simulink model "controller_3dof"  (R2023a)
settings: Solver=FixedStepAuto  StartTime=0.0  StopTime=inf  FixedStep=0.01  RelTol=1e-3  EnableMultiTasking=on
values from neighbouring files (symbols this model uses):
  mf = [22602; 0; -42062;]    [main_3dof.m]
  P0 = diag([P0_ph_meas,P0_th_meas,P0_ps_meas,P0_bias_wp,P0_bias_wq,P0_bias_wr])    [main_3dof.m]
  param = [Ixx;Iyy;Izz;l;k;b;m]    [main_3dof.m]
  Q = diag([q_angle,q_angle,q_angle, q_bias_w_b,q_bias_w_b,q_bias_w_b])    [main_3dof.m]
  R = diag([r_th_meas,r_th_meas,r_ps_meas])    [main_3dof.m]
  Rbody_frd = [cos(angleZ) -sin(angleZ)   0 ... (first row only)    [main_3dof.m]
  Rbody_ned = Rbody_frd*Rfrd_ned    [main_3dof.m]
  Ts_EKF_integr = 0.01    [main_3dof.m]
  Ts_EKF_meas = 0.05    [main_3dof.m]
  Ts_slk = 0.01    [main.m]    (also in main_3dof.m)
  x0EKF = [ph0;th0;ps0;bias_wp0;bias_wq0;bias_wr0]    [main_3dof.m]
undefined symbols (not defined in the file or in its folder): dev, DiscIntNeverNeededParam, Kv, Kx, Main, pwm_output0
libraries: px4Sensorslib x4, px4lib x1, px4uORBlib x1
settings Model: SimulationMode=external  ExtModeTrigDuration=10  Creator=ArriGE66  LastModifiedBy=User
settings SolverCC: PositivePriorityOrder=on
settings OptimizationCC: EnhancedBackFolding=on  PassReuseOutputArgsAs=Individual arguments  ZeroExternalMemoryAtStartup=off  ZeroInternalMemoryAtStartup=off  MaxStackSize=64  OptimizeBlockOrder=speed  DifferentSizesBufferReuse=on  OptimizationCustomize=off  EfficientTunableParamExpr=on
settings DebuggingCC: ParameterTunabilityLossMsg=error
settings HardwareCC: ProdBitPerPointer=32  ProdBitPerSizeT=32  ProdBitPerPtrDiffT=32  ProdLargestAtomicInteger=Long  ProdLargestAtomicFloat=Double  ProdWordSize=32  ProdLongLongMode=on  ProdHWDeviceType=ARM Compatible->ARM Cortex
settings SFSimCC: MATLABDynamicMemAlloc=off  SimTargetLang=C++
settings RTWCC: Description=Embedded Coder  SystemTargetFile=ert.tlc  HardwareBoard=PX4 Cube Orange  TemplateMakefile=ert_default_tmf  Toolchain=GNU Tools for PX4 Autopilots  TargetLang=C++
settings CodeAppCC: ForceParamTrailComments=on  IgnoreCustomStorageClasses=off  OperatorAnnotations=on  SimulinkDataObjDesc=on  SFDataObjDesc=on  InsertBlockDesc=on
settings ERTTargetCC: ExtMode=on  ExtModeTransport=3  ExtModeStaticAlloc=on  ExtModeStaticAllocSize=1024  ExtModeMexFile=ext_xcp  ExtModeMexArgs=1 COM10 3000000  ExtModeIntrfLevel=Level2 - Open

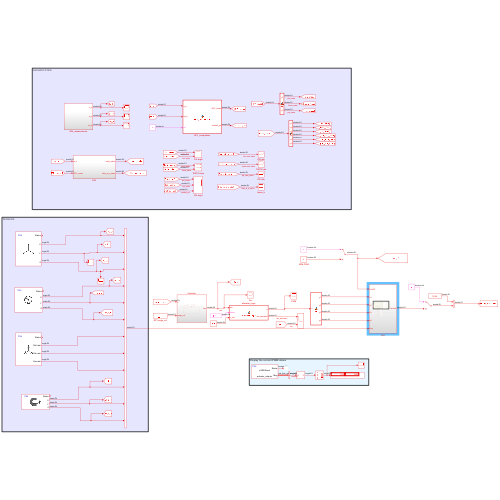
[thumbnail: Simulink's stored preview of the top-level diagram]
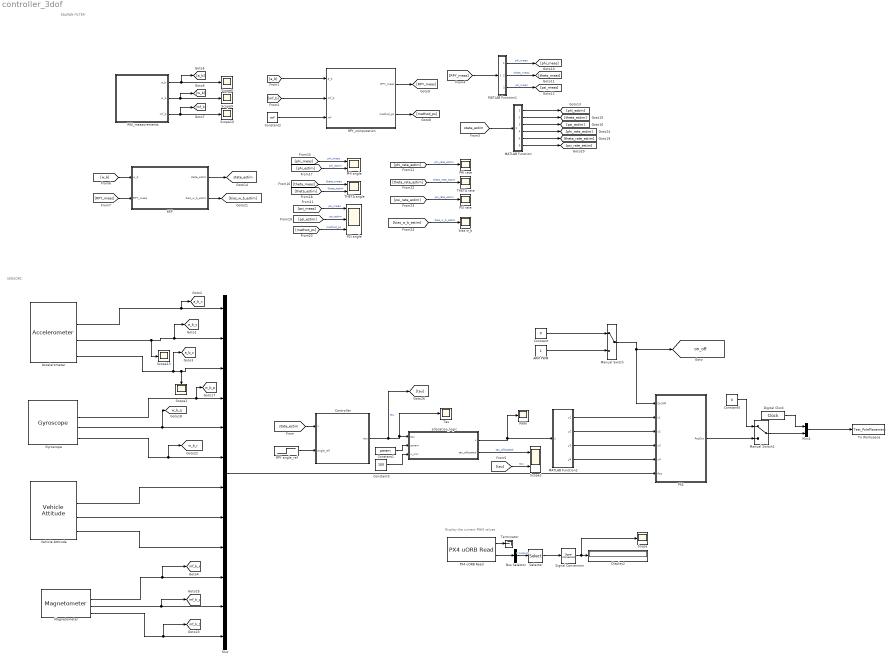
== system controller_3dof ==
  note: KALMAN FILTER
  note: SENSORS
  note: Display the current PWM values
  ARM PWM : Constant  OutDataTypeStr=boolean  SampleTime=0.01
  Accelerometer : px4Sensorslib/Accelerometer  uorbTimeStamp=off  BlockingMode=off  BlockTimeout=1e-3  sampleTime=1/100
  Bus Selector : BusSelector  OutputSignals=output
  Constant : Constant  Value=0  OutDataTypeStr=boolean
  Constant1 : Constant  Value=param
  Constant2 : Constant  Value=mf
  Constant3 : Constant  Value=100  SampleTime=0.01
  Constant5 : Constant  Value=0  OutDataTypeStr=boolean
  Controller : Subsystem
  Digital Clock : DigitalClock  SampleTime=0.01
  Display2 : Display
  EKF : Subsystem
  Gyroscope : px4Sensorslib/Gyroscope  uorbTimeStamp=off  BlockingMode=off  BlockTimeout=1e-3  sampleTime=1/100
  IMU_measurements : Subsystem
  MATLAB Function : MATLAB Function  TreatAsAtomicUnit=on
  MATLAB Function1 : MATLAB Function  TreatAsAtomicUnit=on
  MATLAB Function2 : MATLAB Function  TreatAsAtomicUnit=on
  Magnetometer : px4Sensorslib/Magnetometer  uorbTimeStamp=off  BlockingMode=off  BlockTimeout=1e-3  sampleTime=0.01
  Manual Switch : ManualSwitch
  Manual Switch1 : ManualSwitch
  Mux : Mux  Inputs=12
  Mux1 : Mux  Inputs=2
  PHI angle : Scope  NumInputPorts=2
  PHI rate : Scope
  PSI angle : Scope  NumInputPorts=3
  PSI rate : Scope
  PWM : Scope
  PX4 : Subsystem
  PX4 uORB Read : px4uORBlib/PX4 uORB Read  uORBTopic=actuator_outputs  selectInstance=actuator_outputs  SampleTime=0.01  BlockingMode=off  BlockTimeout=1e-3
  RPY angle_ref : Step  Time=0  After=zeros(3,1)  SampleTime=0.01
  RPY_computation : MATLAB Function  TreatAsAtomicUnit=on
  Scope{,1,8..10,13} (6 alike) : Scope
  Scope2 : Scope  NumInputPorts=2
  Selector : Selector  InputPortWidth=16  IndexOptions=Index vector (dialog)  Indices=[1 2]  OutputSizes=1
  Signal Conversion : SignalConversion  OverrideOpt=off
  THETA angle : Scope  NumInputPorts=2
  THETA rate : Scope
  Tau : Scope
  Terminator : Terminator
  To Workspace : ToWorkspace  VariableName=Test_PolePlacement  SampleTime=-1
      settings: Save2DSignal=2-D array (concatenate along first dimension)
  Vehicle Attitude : px4Sensorslib/Vehicle Attitude  rollRate=on  pitchRate=on  yawRate=on  quaternion=off  uorbTimeStamp=off  BlockingMode=off  BlockTimeout=0.001  sampleTime=1/100
  allocation_logic : MATLAB Function  TreatAsAtomicUnit=on
  bias w_b : Scope
  tag scope: a_b_x=global, a_b_y=global, a_b_z=global, mf_b_x=global, mf_b_y=global, mf_b_z=global, on_off=global, state_estim=global, w_b_p=global, w_b_q=global, w_b_r=global
  wires:
  Bus Selector/1 -> Selector/1  "<output>"
  PX4 uORB Read/1 -> Terminator/1
  Selector/1 -> Signal Conversion/1
  PX4 uORB Read/2 -> Bus Selector/1
  Signal Conversion/1 -> Scope/1, Display2/1
  Vehicle Attitude/3 -> Mux/8
  Vehicle Attitude/2 -> Mux/7
  ARM PWM/1 -> Manual Switch/2
  Constant/1 -> Manual Switch/1
  Gyroscope/4 -> [w_b_r], Mux/6
  Gyroscope/3 -> [w_b_q], Mux/5
  Gyroscope/2 -> [w_b_p], Mux/4
  Accelerometer/2 -> [a_b_x], Mux/1
  Accelerometer/3 -> Scope13/1, [a_b_y], Mux/2
  Accelerometer/4 -> [a_b_z], Mux/3, Scope1/1
  Constant5/1 -> Manual Switch1/1
  Mux1/1 -> To Workspace/1
  Digital Clock/1 -> Mux1/1
  Manual Switch1/1 -> Mux1/2
  Vehicle Attitude/4 -> Mux/9
  Magnetometer/2 -> [mf_b_x], Mux/10
  Magnetometer/3 -> [mf_b_y], Mux/11
  Magnetometer/4 -> [mf_b_z], Mux/12
  MATLAB Function1/2(y2) -> [theta_meas]  "theta_meas"
  [bias_w_b_estim] -> bias w_b/1  "bias_w_b_estim"
  [mf_b] -> RPY_computation/2(mf_b)
  [theta_estim] -> THETA angle/2  "theta_estim"
  MATLAB Function1/1(y1) -> [phi_meas]  "phi_meas"
  [RPY_meas] -> EKF/2(RPY_meas)
  [psi_meas] -> PSI angle/1  "psi_meas"
  [method_ps] -> PSI angle/3  "method_ps"
  IMU_measurements/2(w_b) -> Scope9/1, [w_b]
  [psi_estim] -> PSI angle/2  "psi_estim"
  MATLAB Function1/3(y3) -> [psi_meas]  "psi_meas"
  [RPY_meas] -> MATLAB Function1/1(u)
  [theta_meas] -> THETA angle/1  "theta_meas"
  [phi_rate_estim] -> PHI rate/1  "phi_rate_estim"
  [psi_rate_estim] -> PSI rate/1  "psi_rate_estim"
  [theta_rate_estim] -> THETA rate/1  "theta_rate_estim"
  EKF/1(state_estim) -> [state_estim]
  [phi_estim] -> PHI angle/2  "phi_estim"
  [w_b] -> EKF/1(w_b)
  IMU_measurements/3(mf_b) -> [mf_b], Scope10/1
  Constant2/1 -> RPY_computation/3(mf)
  IMU_measurements/1(a_b) -> [a_b], Scope8/1
  RPY_computation/2(method_ps) -> [method_ps]
  [a_b] -> RPY_computation/1(a_b)
  EKF/2(bias_w_b_estim) -> [bias_w_b_estim]
  [phi_meas] -> PHI angle/1  "phi_meas"
  RPY_computation/1(RPY_meas) -> [RPY_meas]
  Manual Switch/1 -> [on_off], PX4/1(On/Off)
  Mux/1 -> PX4/6(Acq)
  PX4/1(AcqOut) -> Manual Switch1/2
  [state_estim] -> MATLAB Function/1(u)
  MATLAB Function/1(y1) -> [phi_estim]
  MATLAB Function/2(y2) -> [theta_estim]
  MATLAB Function/3(y3) -> [psi_estim]
  MATLAB Function/4(y4) -> [phi_rate_estim]
  MATLAB Function/5(y5) -> [theta_rate_estim]
  MATLAB Function/6(y6) -> [psi_rate_estim]
  MATLAB Function2/4(y4) -> PX4/5(u4)
  MATLAB Function2/3(y3) -> PX4/4(u3)
  MATLAB Function2/2(y2) -> PX4/3(u2)
  MATLAB Function2/1(y1) -> PX4/2(u1)
  allocation_logic/2(tau_allocated) -> Scope2/1  "tau_allocated"
  allocation_logic/1(u) -> PWM/1, MATLAB Function2/1(u)
  Controller/1(tau) -> Tau/1, allocation_logic/1(tau), [tau]  "tau"
  RPY angle_ref/1 -> Controller/2(angle_ref)
  [tau] -> Scope2/2  "tau"
  Constant1/1 -> allocation_logic/2(param)
  [state_estim] -> Controller/1(x)
  Constant3/1 -> allocation_logic/3(u_min)

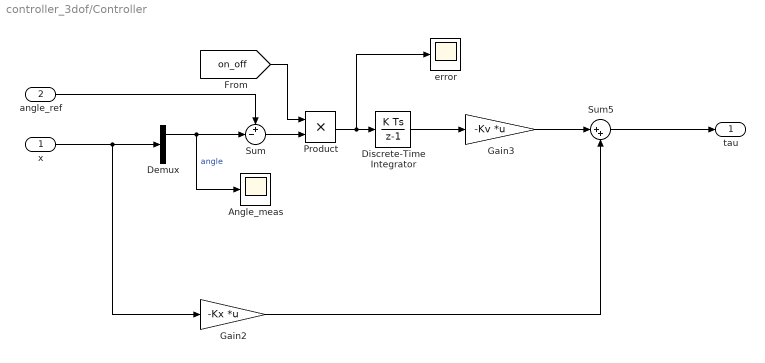
== system controller_3dof/Controller ==
  x : Inport
  angle_ref : Inport  Port=2
  Angle_meas : Scope
  Demux : Demux  Outputs=2
  Discrete-Time Integrator : DiscreteIntegrator  SampleTime=Ts_slk  ICPrevOutput=DiscIntNeverNeededParam  ICPrevScaledInput=DiscIntNeverNeededParam
  Gain2 : Gain  Gain=-Kx  Multiplication=Matrix(K*u)
  Gain3 : Gain  Gain=-Kv  Multiplication=Matrix(K*u)
  Product : Product
  Sum : Sum  Inputs=+-|
  Sum5 : Sum  Inputs=|++
  error : Scope
  tau : Outport
  wires:
  x/1 -> Gain2/1, Demux/1
  Sum5/1 -> tau/1
  angle_ref/1 -> Sum/1
  Discrete-Time Integrator/1 -> Gain3/1
  Gain3/1 -> Sum5/1
  Demux/1 -> Angle_meas/1, Sum/2  "angle"
  Gain2/1 -> Sum5/2
  Sum/1 -> Product/2
  [on_off] -> Product/1
  Product/1 -> error/1, Discrete-Time Integrator/1

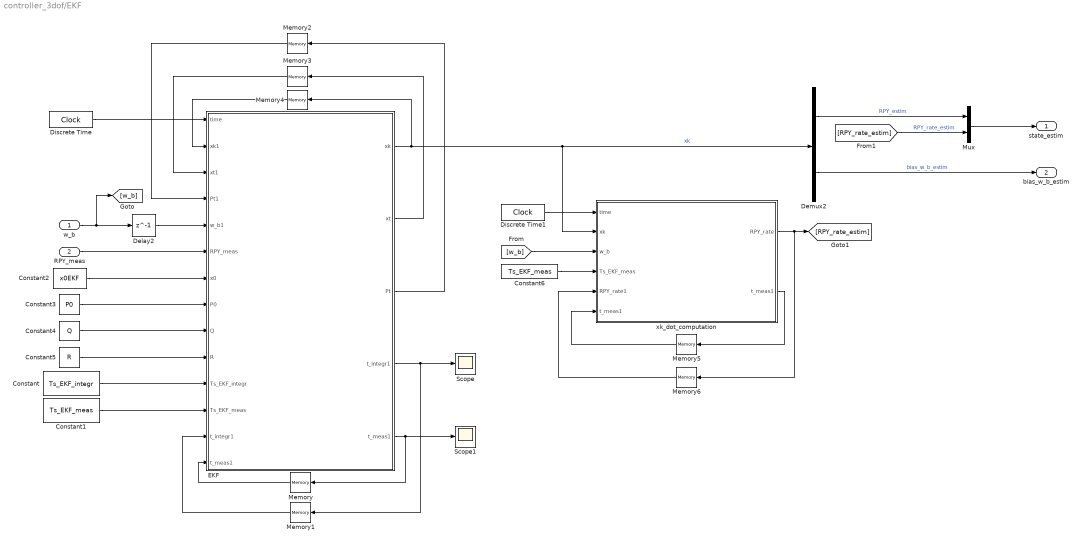
== system controller_3dof/EKF ==
  w_b : Inport
  RPY_meas : Inport  Port=2
  Constant : Constant  Value=Ts_EKF_integr
  Constant1 : Constant  Value=Ts_EKF_meas
  Constant2 : Constant  Value=x0EKF
  Constant3 : Constant  Value=P0
  Constant4 : Constant  Value=Q
  Constant5 : Constant  Value=R
  Constant6 : Constant  Value=Ts_EKF_meas
  Delay2 : Delay  DelayLength=1  SampleTime=Ts_EKF_integr
  Demux2 : Demux  Outputs=2
  Discrete Time : DigitalClock  SampleTime=Ts_slk
  Discrete Time1 : DigitalClock  SampleTime=Ts_slk
  EKF : MATLAB Function  TreatAsAtomicUnit=on
  Memory{,1..6} (7 alike) : Memory
  Mux : Mux  Inputs=2
  Scope : Scope
  Scope1 : Scope
  xk_dot_computation : MATLAB Function  TreatAsAtomicUnit=on
  state_estim : Outport
  bias_w_b_estim : Outport  Port=2
  wires:
  w_b/1 -> Delay2/1, [w_b]
  Constant4/1 -> EKF/9(Q)
  Constant2/1 -> EKF/7(x0)
  Constant5/1 -> EKF/10(R)
  Memory/1 -> EKF/14("t_meas1 ")
  EKF/2(xt) -> Memory3/1
  Memory2/1 -> EKF/4(Pt1)
  EKF/3(Pt) -> Memory2/1
  RPY_meas/1 -> EKF/6(RPY_meas)
  Discrete Time/1 -> EKF/1(time)
  Memory3/1 -> EKF/3(xt1)
  Memory1/1 -> EKF/13("t_integr1 ")
  Constant3/1 -> EKF/8(P0)
  EKF/5(t_meas1) -> Scope1/1, Memory/1
  EKF/4(t_integr1) -> Scope/1, Memory1/1
  Delay2/1 -> EKF/5(w_b1)
  Constant/1 -> EKF/11(Ts_EKF_integr)
  Constant1/1 -> EKF/12(Ts_EKF_meas)
  Memory4/1 -> EKF/2(xk1)
  xk_dot_computation/2(t_meas1) -> Memory5/1
  Memory5/1 -> xk_dot_computation/6("t_meas1 ")
  Memory6/1 -> xk_dot_computation/5(RPY_rate1)
  xk_dot_computation/1(RPY_rate) -> [RPY_rate_estim], Memory6/1
  [w_b] -> xk_dot_computation/3(w_b)
  Discrete Time1/1 -> xk_dot_computation/1(time)
  Demux2/2 -> bias_w_b_estim/1  "bias_w_b_estim"
  Demux2/1 -> Mux/1  "RPY_estim"
  EKF/1(xk) -> xk_dot_computation/2(xk), Demux2/1, Memory4/1  "xk"
  [RPY_rate_estim] -> Mux/2  "RPY_rate_estim"
  Mux/1 -> state_estim/1
  Constant6/1 -> xk_dot_computation/4(Ts_EKF_meas)

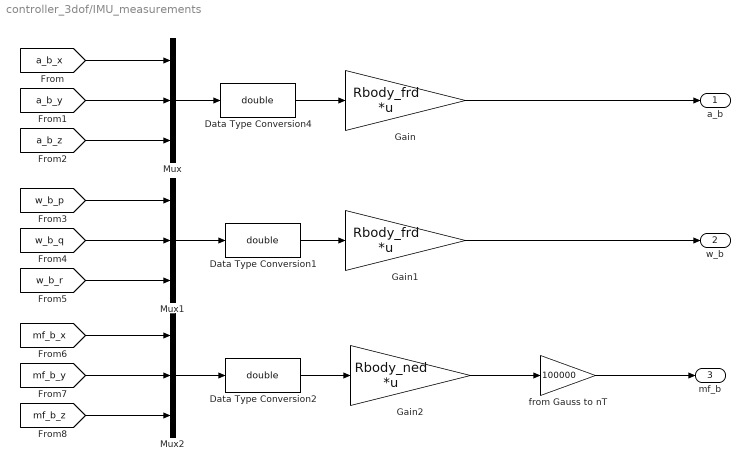
== system controller_3dof/IMU_measurements ==
  Data Type Conversion1 : DataTypeConversion  OutDataTypeStr=double  SaturateOnIntegerOverflow=off  RndMeth=Floor
  Data Type Conversion2 : DataTypeConversion  OutDataTypeStr=double  SaturateOnIntegerOverflow=off  RndMeth=Floor
  Data Type Conversion4 : DataTypeConversion  OutDataTypeStr=double  SaturateOnIntegerOverflow=off  RndMeth=Floor
  Gain : Gain  Gain=Rbody_frd  Multiplication=Matrix(K*u) (u vector)
  Gain1 : Gain  Gain=Rbody_frd  Multiplication=Matrix(K*u) (u vector)
  Gain2 : Gain  Gain=Rbody_ned  Multiplication=Matrix(K*u) (u vector)
  Mux : Mux  Inputs=3
  Mux1 : Mux  Inputs=3
  Mux2 : Mux  Inputs=3
  from Gauss to nT : Gain  Gain=100000
  a_b : Outport
  w_b : Outport  Port=2
  mf_b : Outport  Port=3
  wires:
  Gain2/1 -> from Gauss to nT/1
  Mux2/1 -> Data Type Conversion2/1
  [a_b_x] -> Mux/1
  [a_b_y] -> Mux/2
  [a_b_z] -> Mux/3
  Mux/1 -> Data Type Conversion4/1
  Mux1/1 -> Data Type Conversion1/1
  [w_b_p] -> Mux1/1
  [w_b_r] -> Mux1/3
  [w_b_q] -> Mux1/2
  [mf_b_x] -> Mux2/1
  [mf_b_z] -> Mux2/3
  [mf_b_y] -> Mux2/2
  Gain/1 -> a_b/1
  Gain1/1 -> w_b/1
  from Gauss to nT/1 -> mf_b/1
  Data Type Conversion4/1 -> Gain/1
  Data Type Conversion1/1 -> Gain1/1
  Data Type Conversion2/1 -> Gain2/1

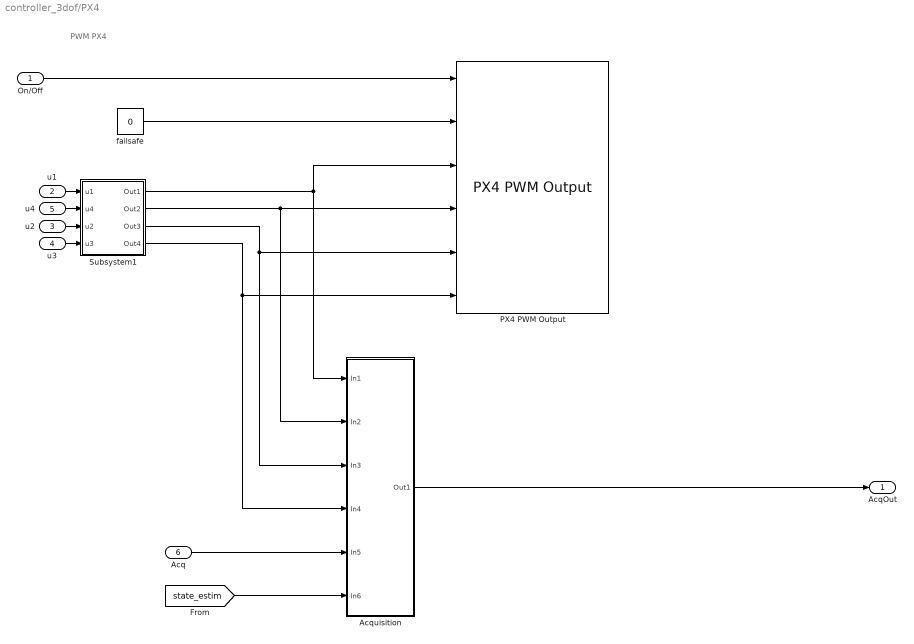
== system controller_3dof/PX4 ==
  note: PWM PX4
  On/Off : Inport
  u1 : Inport  Port=2
  u2 : Inport  Port=3
  u3 : Inport  Port=4
  u4 : Inport  Port=5
  Acq : Inport  Port=6
  Acquisition : Subsystem
  PX4 PWM Output : px4lib/PX4 PWM Output  pwmDevice=Main (/dev/pwm_output0)  pwmChannel1_=on  pwmChannel2_=on  pwmChannel3_=on  pwmChannel4_=on  pwmChannel5_=off  pwmChannel6_=off  pwmChannel7_=off  pwmChannel8_=off  forceTerminateFailsafe=off  outputErrorStatus=on
  Subsystem1 : Subsystem
  failsafe : Constant  Value=0  OutDataTypeStr=boolean  SampleTime=0.01
  AcqOut : Outport
  wires:
  failsafe/1 -> PX4 PWM Output/2
  Subsystem1/2(Out2) -> Acquisition/2(In2), PX4 PWM Output/4
  Subsystem1/4(Out4) -> Acquisition/4(In4), PX4 PWM Output/6
  Subsystem1/3(Out3) -> Acquisition/3(In3), PX4 PWM Output/5
  Subsystem1/1(Out1) -> Acquisition/1(In1), PX4 PWM Output/3
  Acq/1 -> Acquisition/5(In5)
  On/Off/1 -> PX4 PWM Output/1
  u4/1 -> Subsystem1/2(u4)
  Acquisition/1(Out1) -> AcqOut/1
  u1/1 -> Subsystem1/1(u1)
  u2/1 -> Subsystem1/3(u2)
  u3/1 -> Subsystem1/4(u3)
  [state_estim] -> Acquisition/6(In6)

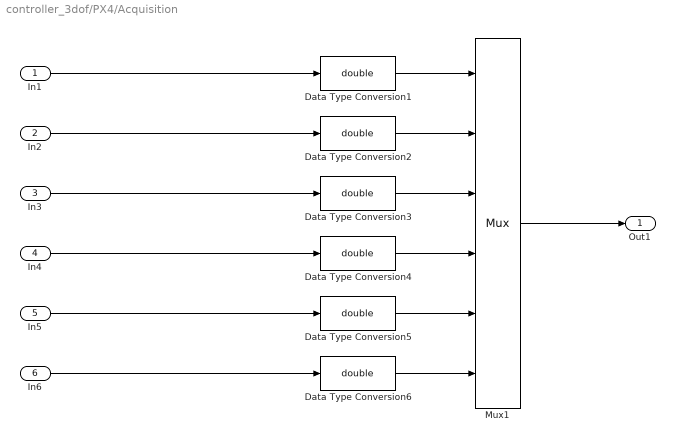
== system controller_3dof/PX4/Acquisition ==
  In1 : Inport
  In2 : Inport  Port=2
  In3 : Inport  Port=3
  In4 : Inport  Port=4
  In5 : Inport  Port=5
  In6 : Inport  Port=6
  Data Type Conversion{1..6} (6 alike) : DataTypeConversion  OutDataTypeStr=double  SaturateOnIntegerOverflow=off  RndMeth=Floor
  Mux1 : Mux  Inputs=6
      settings: DisplayOption=signals
  Out1 : Outport
  wires:
  In2/1 -> Data Type Conversion2/1
  Data Type Conversion1/1 -> Mux1/1
  Data Type Conversion3/1 -> Mux1/3
  Data Type Conversion5/1 -> Mux1/5
  Data Type Conversion4/1 -> Mux1/4
  Data Type Conversion2/1 -> Mux1/2
  Data Type Conversion6/1 -> Mux1/6
  In3/1 -> Data Type Conversion3/1
  In6/1 -> Data Type Conversion6/1
  Mux1/1 -> Out1/1
  In5/1 -> Data Type Conversion5/1
  In1/1 -> Data Type Conversion1/1
  In4/1 -> Data Type Conversion4/1

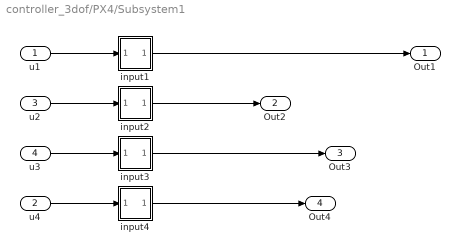
== system controller_3dof/PX4/Subsystem1 ==
  u1 : Inport
  u4 : Inport  Port=2
  u2 : Inport  Port=3
  u3 : Inport  Port=4
  input1 : Subsystem
  input2 : Subsystem
  input3 : Subsystem
  input4 : Subsystem
  Out1 : Outport
  Out2 : Outport  Port=2
  Out3 : Outport  Port=3
  Out4 : Outport  Port=4
  wires:
  u2/1 -> input2/1(In1)
  u1/1 -> input1/1(In1)
  input1/1(Out1) -> Out1/1
  u4/1 -> input4/1(In1)
  input4/1(Out1) -> Out4/1
  input2/1(Out1) -> Out2/1
  u3/1 -> input3/1(In1)
  input3/1(Out1) -> Out3/1

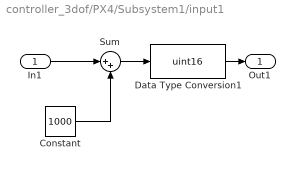
== system controller_3dof/PX4/Subsystem1/input1 ==
  In1 : Inport
  Constant : Constant  Value=1000  SampleTime=0.01
  Data Type Conversion1 : DataTypeConversion  OutDataTypeStr=uint16  SaturateOnIntegerOverflow=off  RndMeth=Floor
  Sum : Sum  Inputs=|++
  Out1 : Outport
  wires:
  Sum/1 -> Data Type Conversion1/1
  In1/1 -> Sum/1
  Constant/1 -> Sum/2
  Data Type Conversion1/1 -> Out1/1

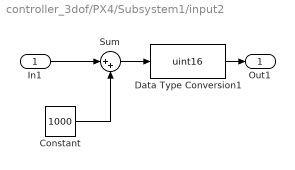
== system controller_3dof/PX4/Subsystem1/input2 ==
  In1 : Inport
  Constant : Constant  Value=1000  SampleTime=0.01
  Data Type Conversion1 : DataTypeConversion  OutDataTypeStr=uint16  SaturateOnIntegerOverflow=off  RndMeth=Floor
  Sum : Sum  Inputs=|++
  Out1 : Outport
  wires:
  Sum/1 -> Data Type Conversion1/1
  In1/1 -> Sum/1
  Constant/1 -> Sum/2
  Data Type Conversion1/1 -> Out1/1

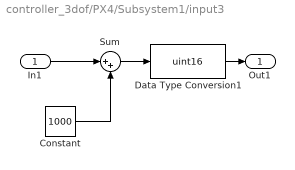
== system controller_3dof/PX4/Subsystem1/input3 ==
  In1 : Inport
  Constant : Constant  Value=1000  SampleTime=0.01
  Data Type Conversion1 : DataTypeConversion  OutDataTypeStr=uint16  SaturateOnIntegerOverflow=off  RndMeth=Floor
  Sum : Sum  Inputs=|++
  Out1 : Outport
  wires:
  Sum/1 -> Data Type Conversion1/1
  In1/1 -> Sum/1
  Constant/1 -> Sum/2
  Data Type Conversion1/1 -> Out1/1

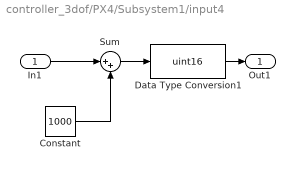
== system controller_3dof/PX4/Subsystem1/input4 ==
  In1 : Inport
  Constant : Constant  Value=1000  SampleTime=0.01
  Data Type Conversion1 : DataTypeConversion  OutDataTypeStr=uint16  SaturateOnIntegerOverflow=off  RndMeth=Floor
  Sum : Sum  Inputs=|++
  Out1 : Outport
  wires:
  Sum/1 -> Data Type Conversion1/1
  In1/1 -> Sum/1
  Constant/1 -> Sum/2
  Data Type Conversion1/1 -> Out1/1

== matlab function controller_3dof/allocation_logic ==
  data: tau input; u output; param input; tau_allocated output; u_min input
function [u, tau_allocated] = allocation_logic(tau,param, u_min)
% Allocation Logic Block: computes the corresponding control command
% u = [u1,u2,u3,u4] given the torque command tau = [tau_phi, tau_theta, tau_phi]

% control command limits
%%u_min = 100;
u_max = 1000;

l = param(4,1);
k = param(5,1);
b = param(6,1);

% [tau_ph; tau_th; tau_ps]' = Mtau_u * [u1;u2;u3;u4]
Mtau_u = [0      0       l*k     -l*k;
          -l*k   l*k     0       0;
          -b     -b      b       b;];
Minv = Mtau_u'*inv(Mtau_u*Mtau_u');
up = Minv*tau;
un = zeros(4,1);
if min(up(:)) < u_min 
    un = ones(4,1)*(u_min - min(up(:)));
end
u = up+un;
for i = 1:1:4
    if u(i,1) > u_max
        u(i,1) = u_max;
    end
end
 tau_allocated = Mtau_u*u;

== matlab function controller_3dof/MATLAB Function1 ==
  data: u input; y1 output; y2 output; y3 output
function [y1,y2,y3] = fcn(u)

y1 = u(1);
y2 = u(2);
y3 = u(3);

== matlab function controller_3dof/MATLAB Function ==
  data: u input; y1 output; y2 output; y3 output; y4 output; y5 output; y6 output
function [y1,y2,y3,y4,y5,y6] = fcn(u)

y1 = u(1);
y2 = u(2);
y3 = u(3);
y4 = u(4);
y5 = u(5);
y6 = u(6);

== matlab function controller_3dof/MATLAB Function2 ==
  data: u input; y1 output; y2 output; y3 output; y4 output
function [y1,y2,y3,y4] = fcn(u)

y1 = u(1);
y2 = u(2);
y3 = u(3);
y4 = u(4);

== matlab function controller_3dof/RPY_computation ==
  data: a_b input; mf_b input; RPY_meas output; mf input; method_ps output
function [RPY_meas,method_ps]   = RPY_computation(a_b,mf_b,mf)
% description:
% - a_b             = measured linear acceleration in body-frame
% - w_b             = measured angular velocity in body-frame
% - mf_b            = measured magnetic field in body-frame
% - mf              = measured magnetic field in body-inertia
% - a_b_disturbe    = linear velocity measurement-noise
% - w_b_disturbe    = angular velocity measurement-noise
% - mf_b_disturbe   = magnetic field measurement-noise

% -------------------------------------------------------------------------------------------
% observation: the following computation works only if the angles
% phi,theta,psy are withing angles (-pi/2,+pi/2) (this is an open set, pi/2 is excluded)
% -------------------------------------------------------------------------------------------

a_b = -1*a_b;       % need to adjust the sign to use atan2() function correctly
mf_u = mf(3,1);     % magnetic field in up direction (z-dir in inertia frame)

% phi computation
ph_meas = atan2(a_b(2), a_b(3));
sph = sin(ph_meas);
cph = cos(ph_meas);

% theta computation
th_meas = atan2(-a_b(1), (a_b(2)*sph + a_b(3)*cph));
sth = sin(th_meas);
cth = cos(th_meas);

% psi computation
if abs(sin(th_meas)) > 0.1  % sin(th) != 0 
    method_ps = 1;
    ps_meas_numerator   = (sth*cph*mf_b(2) - sth*sph*mf_b(3))/(-sth);       % don't modify
    ps_meas_denominator = (-sph*mf_b(2) - cph*mf_b(3) + cth*mf_u)/(-sth);   % don't modify
    ps_meas = atan2(ps_meas_numerator, ps_meas_denominator);
else                        % sin(th) == 0
    method_ps = 2;
    ps_meas_numerator   = (mf_b(2) - cth*sph*mf_u)*(-cth);
    ps_meas_denominator = cph*mf_b(1);
    ps_meas = atan2(ps_meas_numerator, ps_meas_denominator);
end
RPY_meas = [ph_meas;th_meas;ps_meas];

== matlab function controller_3dof/EKF/EKF ==
  data: time input; xk1 input; xt1 input; Pt1 input; w_b1 input; RPY_meas input; x0 input; P0 input; Q input; R input; Ts_EKF_integr input; Ts_EKF_meas input; xk output; t_integr1 input; t_meas1 input; xt output; Pt output; t_integr1 output; t_meas1 output
function [xk,xt,Pt,t_integr1,t_meas1] = EKF(time,xk1,xt1,Pt1,w_b1,RPY_meas,x0,P0,Q,R,Ts_EKF_integr,Ts_EKF_meas,t_integr1,t_meas1)

if time == 0
    xk = x0;
    xt = x0;
    Pt = P0;
    t_integr1 = 0;
    t_meas1 = 0;
elseif time - t_integr1 >= Ts_EKF_integr
    wp          =       w_b1(1,1);        % p-dir of angular velocity w
    wq          =       w_b1(2,1);        % q-dir of angular velocity w
    wr          =       w_b1(3,1);        % r-dir of angular velocity w

    phi         =       xt1(1,1);         %  roll angle (rad)
    theta       =       xt1(2,1);         %  pitch angle (rad)
    psi         =       xt1(3,1);         %  yaw angle (rad)  
    bias_wp     =       xt1(4,1);         % bias of p-dir of angular velocity w
    bias_wq     =       xt1(5,1);         % bias of q-dir of angular velocity w
    bias_wr     =       xt1(6,1);         % bias of r-dir of angular velocity w

    cph         =       cos(phi);
    cth         =       cos(theta);
    cps         =       cos(psi);
    sph         =       sin(phi);
    sth         =       sin(theta);
    sps         =       sin(psi);
    tth         =       sth/cth;

    % integration step
    t_integr1 = time;
    Mf = [1,    sph*tth,    cph*tth,    0,  0,  0;
          0,    cph,        -sph,       0,  0,  0;
          0,    sph/cth,    cph/cth,    0,  0,  0;
          0,    0,          0,          1,  0,  0;
          0,    0,          0,          0,  1,  0;
          0,    0,          0,          0,  0,  1;];
    Z1 = [wp-bias_wp; wq-bias_wq; wr-bias_wr; bias_wp; bias_wq; bias_wr;];
    f = Mf*Z1;
    xt = xt1 + Ts_EKF_integr*f;

    A1 = [cph*tth*(wq-bias_wq)-sph*tth*(wr-bias_wr),(sph*(wq-bias_wq)+cph*(wr-bias_wr))/cth^2,  0,  -1, -sph*tth,   -cph*tth;];
    A2 = [-sph*(wq-bias_wq)-cph*(wr-bias_wr),   0,  0,  0,  -cph,   sph;];
    A3 = [cph*(wq-bias_wq)/cth-sph*(wr-bias_wr)/cth, (sth/cth^2)*(sph*(wq-bias_wq)+cph*(wr-bias_wr)),   0,  0,  -sph/cth,   -cph/cth;];
    A4 = [0,    0,  0,  1,  0,  0;];
    A5 = [0,    0,  0,  0,  1,  0;];
    A6 = [0,    0,  0,  0,  0,  1;];
    At1 = [A1; A2; A3; A4; A5; A6;];
    Pt = Pt1 + Ts_EKF_integr*(At1*Pt1 + Pt1*At1' + Q);

    % measurement step
    if time - t_meas1 >= Ts_EKF_meas
        t_meas1 = time;
        Ck = [eye(3),zeros(3,3)];
        Lk = Pt*Ck'/(Ck*Pt*Ck' + R);
        xk = xt + Lk*(RPY_meas - Ck*xt);
        Pk = (eye(6) - Lk*Ck)*Pt;

        xt = xk;    % becomes the new xt1
        Pt = Pk;    % becomes the new Pt1
    else
        xk = xk1;    % xk1
    end
else
    xk = xt1;
    xt = xt1;
    Pt = Pt1;
end
end

== matlab function controller_3dof/EKF/xk_dot_computation ==
  data: time input; xk input; w_b input; Ts_EKF_meas input; RPY_rate1 input; RPY_rate output; t_meas1 input; t_meas1 output
function [RPY_rate,t_meas1] = xk_dot_computation(time,xk,w_b,Ts_EKF_meas,RPY_rate1,t_meas1)
RPY_rate = zeros(3,1);
if time == 0
    t_meas1 = 0;
end
if time - t_meas1 >= Ts_EKF_meas || time == 0
    wp          =       w_b(1,1);        % p-dir of angular velocity w
    wq          =       w_b(2,1);        % q-dir of angular velocity w
    wr          =       w_b(3,1);        % r-dir of angular velocity w

    phi         =       xk(1,1);         %  roll angle (rad)
    theta       =       xk(2,1);         %  pitch angle (rad)
    psi         =       xk(3,1);         %  yaw angle (rad)  
    bias_wp     =       xk(4,1)*0;         % bias of p-dir of angular velocity w
    bias_wq     =       xk(5,1)*0;         % bias of q-dir of angular velocity w
    bias_wr     =       xk(6,1)*0;         % bias of r-dir of angular velocity w

    cph         =       cos(phi);
    cth         =       cos(theta);
    cps         =       cos(psi);
    sph         =       sin(phi);
    sth         =       sin(theta);
    sps         =       sin(psi);
    tth         =       sth/cth;

    % integration step
    t_meas1 = time;
    W_eta = [1,    sph*tth,    cph*tth;
             0,    cph,        -sph;
             0,    sph/cth,    cph/cth;];
    w_b_corrected = [wp-bias_wp; wq-bias_wq; wr-bias_wr;];
    RPY_rate = W_eta*w_b_corrected;
else
    RPY_rate = RPY_rate1;
end
end
